simulink model "ims_Build5pt1h_tj"  (R2020b)
settings: Solver=FixedStepDiscrete  StartTime=0.0  StopTime=180  FixedStep=fem.Ts  RelTol=1e-4
InitFcn:
  | %
  | % Initialization callback function
  | %
  | 
  | try
  |    fprintf('\n New GMT IMS version!\n');
  | 
  |    % Get Simulink model directory
  |    [filepath,name,ext] = fileparts(which(bdroot));
  | 
  |    if ~strcmp(filepath,pwd)
  |       fprintf('\n Changing current directory to \n %s \n',filepath);
  |       cd(filepath);
  |    end
  | 
  |    %
  |    if(~exist('IMLoads','var'))
  |        warning('Simulation model assumes wind load is loaded...');
  |    end
  | catch
  |    warning('Running the InitFcn from puSimulate script');
  | end
values from neighbouring files (symbols this model uses):
  az = zeros(N,1)    [eval_trajectories.m]
  az_ff_en = 0    [load_IMS_5pt1g_tj.m]    (also in load_IMS_5pt1h_tj.m)
  el = az    [eval_trajectories.m]
  el_ff_en = 0    [load_IMS_5pt1g_tj.m]    (also in load_IMS_5pt1h_tj.m)
  fem =     [controls_5pt1g1K_z00_llTT_oad.mat]    (also in controls_5pt1g1K_z30_llTT_oad.mat)
  FEM_Ts = 1/1e3    (= 0.001)    [load_IMS_5pt1g_tj.m]    (also in load_IMS_5pt1h_tj.m)
  gir = az    [eval_trajectories.m]
  gir_ff_en = 0    [load_IMS_5pt1g_tj.m]    (also in load_IMS_5pt1h_tj.m)
  H_tj = tf(1,[2*pi*0.1, 1])    [eval_trajectories.m]    (also in load_IMS_5pt1g_tj.m = c2d(Htjf,FEM_Ts, 'foh'); load_IMS_5pt1h_tj.m = c2d(Htjf,FEM_Ts, 'foh'))
  Hkin = [-8.71000900827 -2.52558087914e-07 3.42467822122e-06 8.28158913389e-05 0.235170938796 0.971955089687 -8.71000882983 -2.56988849003e-07 -1.09343631703e-06 2.92892772526e-07 0.235169927865 0.971955316524 ... (252 elements, 84x3)]    [controls_5pt1g1K_z00_llTT_oad.mat]    (also in controls_5pt1g1K_z30_llTT_oad.mat = [-5.06628586419 -1.02311476859e-06 3.2470665042e-06 5.646393; load_IMS_5pt1g_tj.m = [HkinAZ_sim, HkinEL_sim, zeros(84,1)]; load_IMS_5pt1h_tj.m = [HkinAZ_sim, HkinEL_sim, zeros(84,1)])
  Hkin_pmt = [pmt1;pmt2]*Hkin_pmtnodes    [eval_tjs.m]    (also in eval_tjs_rtf_variants.m; load_IMS_5pt1g_tj.m = [HkinAZ_00_pmt, HkinEL_00_pmt, zeros(21,1)]; load_IMS_5pt1h_tj.m = [HkinAZ_00_pmt, HkinEL_00_pmt, zeros(21,1)])
  m1olf_en = 0    [load_IMS_5pt1g_tj.m]    (also in load_IMS_5pt1h_tj.m)
  m1sys =     [controls_5pt1g1K_z00_llTT_oad.mat]    (also in controls_5pt1g1K_z30_llTT_oad.mat)
  m2_pos_en = 0    [load_IMS_5pt1g_tj.m]    (also in load_IMS_5pt1h_tj.m)
  m2pos =     [controls_5pt1g1K_z00_llTT_oad.mat]    (also in controls_5pt1g1K_z30_llTT_oad.mat)
  m2pzt =     [controls_5pt1g1K_z00_llTT_oad.mat]    (also in controls_5pt1g1K_z30_llTT_oad.mat)
  m2PZT_en = 0    [load_IMS_5pt1g_tj.m]    (also in load_IMS_5pt1h_tj.m)
  mntFBc_en = 1    [load_IMS_5pt1g_tj.m]    (also in load_IMS_5pt1h_tj.m)
  mount =     [controls_5pt1g1K_z00_llTT_oad.mat]    (also in controls_5pt1g1K_z30_llTT_oad.mat; eval_tjs.m = mountY)
  om2 = (2*pi*eigenfrequencies).^2    [load_IMS_5pt1g_tj.m]    (also in load_IMS_5pt1h_tj.m)
  PG = zeros(length(om2),6)    [load_IMS_5pt1g_tj.m]    (also in load_IMS_5pt1h_tj.m)
  phiB = Phim(indDesInputs,:)'    [load_IMS_5pt1g_tj.m]    (also in load_IMS_5pt1h_tj.m)
  phiC = Phi(indDesOutputs,:)    [load_IMS_5pt1g_tj.m]    (also in load_IMS_5pt1h_tj.m)
  pmt1 = dlmread(pmt1_fname,',',[14,3,27,302])    [eval_tjs.m]    (also in eval_tjs_rtf_variants.m; load_IMS_5pt1g_tj.m; load_IMS_5pt1h_tj.m)
  pmt2 = dlmread(pmt2_fname,',',[14,3,10,302])    [eval_tjs.m]    (also in eval_tjs_rtf_variants.m; load_IMS_5pt1g_tj.m; load_IMS_5pt1h_tj.m)
  Psi_ss = gainMatrix(indDesOutputs,indDesInputs) - K_ss    [load_IMS_5pt1g_tj.m]    (also in load_IMS_5pt1h_tj.m)
  Psi_ssTs = 1/1000    (= 0.001)    [load_IMS_5pt1g_tj.m]    (also in load_IMS_5pt1h_tj.m)
  twice_zom = adjDamp*twice_zom    [load_IMS_5pt1g_tj.m]    (also in load_IMS_5pt1h_tj.m)
undefined symbols (not defined in the file or in its folder): az2M1, az2M2, DiscIntNeverNeededParam, el2M1, el2M2, magnitude
libraries: ims_block_library x20, simulink x1
(part 3 of 3)

== system ims_Build5pt1h_tj/Mount_Drv_PDR2021/ODC CT LUGRE Fr model/Friction/Friction Gir/g(v)/gs ==
  v : Inport
  Enable : EnablePort
  Divide : Product  Inputs=**
  Gain : Gain  Gain=1/vs
  Math Function : Math  SignedPower=on  SaturateOnIntegerOverflow=on
  Math Function1 : Math  Operator=magnitude^2  SignedPower=on  SaturateOnIntegerOverflow=on
  Unary Minus : UnaryMinus
  gs : Constant  Value=(Ts-Tc)/sigma0
  gs(v) : Outport
  wires:
  Math Function/1 -> Divide/1
  gs/1 -> Divide/2
  Math Function1/1 -> Unary Minus/1
  Unary Minus/1 -> Math Function/1
  Gain/1 -> Math Function1/1
  v/1 -> Gain/1
  Divide/1 -> gs(v)/1

== system ims_Build5pt1h_tj/Mount_Drv_PDR2021/Parasitic torques model /Subsystem/Parasitic Torques/Parasitic GIR/Cogging ==
  Po : Inport
  CogAmp : Constant  Value=cog_amp
  CogSpatFreq : Constant  Value=cog_sfr
  Product1 : Product  RndMeth=Zero
  Product2 : Product  RndMeth=Zero
  Trigonometric Function : Trigonometry
  T_cog : Outport
  wires:
  Product1/1 -> Trigonometric Function/1
  CogSpatFreq/1 -> Product1/2
  CogAmp/1 -> Product2/2
  Trigonometric Function/1 -> Product2/1
  Po/1 -> Product1/1
  Product2/1 -> T_cog/1

== system ims_Build5pt1h_tj/Mount_Drv_PDR2021/Parasitic torques model /Subsystem/Parasitic Torques/Parasitic GIR/Emf ==
  To : Inport
  Po : Inport  Port=2
  EmfAmpFactor : Constant  Value=emf_ampFact
  EmfSpatFreq : Constant  Value=emf_sfr
  Product1 : Product  RndMeth=Zero
  Product2 : Product  Inputs=3  RndMeth=Zero
  Trigonometric Function : Trigonometry
  T_emf : Outport
  wires:
  Product1/1 -> Trigonometric Function/1
  EmfSpatFreq/1 -> Product1/2
  EmfAmpFactor/1 -> Product2/2
  Trigonometric Function/1 -> Product2/1
  Po/1 -> Product1/1
  Product2/1 -> T_emf/1
  To/1 -> Product2/3
